simulink model "PIZANO_LAB5_part1"  (Simulink 10.0)
settings: Solver=FixedStepAuto  StartTime=0.0  StopTime=6  FixedStep=0.001  RelTol=1e-3
libraries: simulink x1
settings Model: Creator=XxaemaeThxX  LastModifiedBy=XxaemaeThxX
settings DataIOCC: SaveFormat=Dataset  ReturnWorkspaceOutputs=on
settings OptimizationCC: LifeSpan=auto
settings DebuggingCC: UnderspecifiedInitializationDetection=Simplified  MergeDetectMultiDrivingBlocksExec=error  SFUnexpectedBacktrackingDiag=error  SFNoUnconditionalDefaultTransitionDiag=error  SFExecutionAtInitializationDiag=warning  ArithmeticOperatorsInVariantConditions=error
settings HardwareCC: ProdBitPerPointer=64  ProdBitPerSizeT=64  ProdBitPerPtrDiffT=64  ProdLargestAtomicFloat=Float  ProdIntDivRoundTo=Zero  ProdEndianess=LittleEndian  ProdWordSize=64  ProdHWDeviceType=Intel->x86-64 (Windows64)
settings ModelReferenceCC: PropagateSignalLabelsOutOfModel=on
settings SFSimCC: SimUseLocalCustomCode=on  CustomCodeUndefinedFunction=FilterOut
settings RTWCC: RTWUseLocalCustomCode=on
settings CodeAppCC: StateflowObjectComments=off
settings GRTTargetCC: TargetLangStandard=C99 (ISO)  CombineOutputUpdateFcns=on  GRTInterface=off
settings ConfigComp: CovMetricSettings=dwe  CovHtmlReporting=off  CovSaveCumulativeToWorkspaceVar=off  CovSaveSingleToWorkspaceVar=off

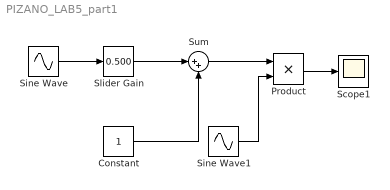
== system PIZANO_LAB5_part1 ==
  Constant : Constant
  Product : Product  RndMeth=Zero
  Scope1 : Scope
  Sine Wave : Sin  Frequency=5  SampleTime=0
  Sine Wave1 : Sin  Amplitude=2  Frequency=200  SampleTime=0
  Slider Gain : simulink/Math Operations/Slider Gain  gain=0.500  low=0  high=2
  Sum : Sum  Inputs=|++
  wires:
  Sine Wave1/1 -> Product/2
  Sum/1 -> Product/1
  Sine Wave/1 -> Slider Gain/1
  Constant/1 -> Sum/2
  Product/1 -> Scope1/1
  Slider Gain/1 -> Sum/1
